simulink model "comparison_simulator"  (R2025b)
settings: Solver=VariableStepAuto  StartTime=0.0  StopTime=1000  RelTol=1e-3
values from neighbouring files (symbols this model uses):
  FO_PI = minreal(kp_FO + kp_FO*ki_FO*tf(1,[1 0])*s_alfa1, 0.1)    [controller_design.m]
  Hc_GT = minreal((1/H_p) * (Ho_GT / (1-Ho_GT)))    [controller_design.m]
  Hc_PI = minreal(ki_PI * (1 + tf(1, [Ti_PI 0])))    [controller_design.m]
  Rc_IMC = minreal(Hc_IMC / minreal(1 - Hc_IMC * H_p))    [controller_design.m]
undefined symbols (not defined in the file or in its folder): MAP_model, paramGrecoMAP
libraries: slpidlib x1
settings Model: Creator=ciuba  LastModifiedBy=ciuba

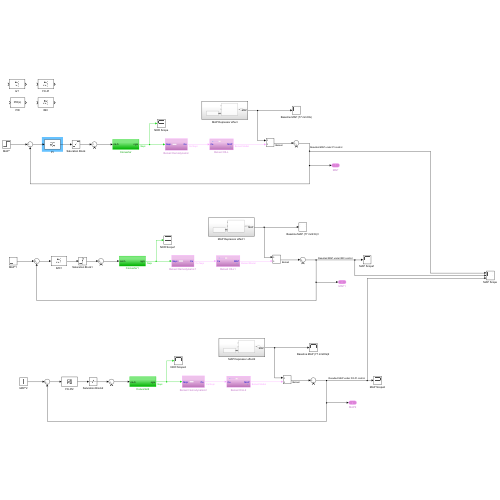
[thumbnail: Simulink's stored preview of the top-level diagram]
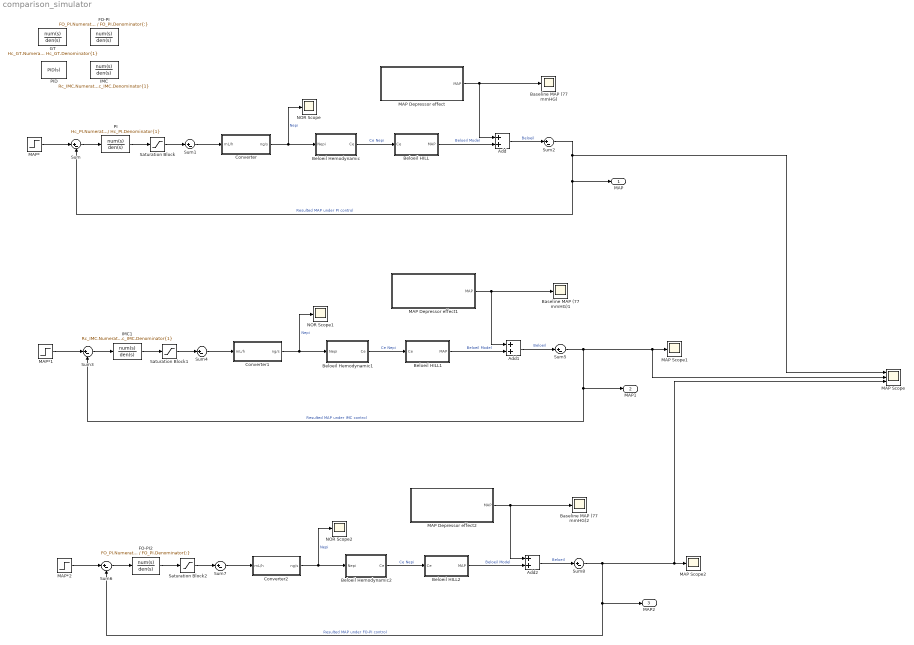
== system comparison_simulator ==
  Add : Sum
  Add1 : Sum
  Add2 : Sum
  Baseline MAP (77 mmHG) : Scope
      settings: ActiveDisplayYMinimum=-1  ActiveDisplayYMaximum=1  DataLoggingVariableName=ScopeData6
  Baseline MAP (77 mmHG)1 : Scope
      settings: ActiveDisplayYMinimum=-1  ActiveDisplayYMaximum=1
  Baseline MAP (77 mmHG)2 : Scope
      settings: ActiveDisplayYMinimum=-1  ActiveDisplayYMaximum=1  DataLoggingVariableName=ScopeData3
  Beloeil HILL : Subsystem
  Beloeil HILL1 : Subsystem
  Beloeil HILL2 : Subsystem
  Beloeil Hemodynamic : Subsystem
  Beloeil Hemodynamic1 : Subsystem
  Beloeil Hemodynamic2 : Subsystem
  Converter : Subsystem
  Converter1 : Subsystem
  Converter2 : Subsystem
  FO-PI : TransferFcn  Numerator=FO_PI.Numerator{:}  Denominator=FO_PI.Denominator{:}
  FO-PI2 : TransferFcn  Numerator=FO_PI.Numerator{:}  Denominator=FO_PI.Denominator{:}
  GT : TransferFcn  Numerator=Hc_GT.Numerator{1}  Denominator=Hc_GT.Denominator{1}
  IMC : TransferFcn  Numerator=Rc_IMC.Numerator{1}  Denominator=Rc_IMC.Denominator{1}
  IMC1 : TransferFcn  Numerator=Rc_IMC.Numerator{1}  Denominator=Rc_IMC.Denominator{1}
  MAP Depressor effect : Subsystem
  MAP Depressor effect1 : Subsystem
  MAP Depressor effect2 : Subsystem
  MAP Scope : Scope  NumInputPorts=3
      settings: ActiveDisplayYMinimum=75.156439251217392  ActiveDisplayYMaximum=93.5920467390435  DataLoggingVariableName=ScopeData4
  MAP Scope1 : Scope
      settings: ActiveDisplayYMinimum=75.156363433588581  ActiveDisplayYMaximum=93.592729097702758
  MAP Scope2 : Scope
      settings: ActiveDisplayYMinimum=75.156363433588581  ActiveDisplayYMaximum=93.592729097702758  DataLoggingVariableName=ScopeData5
  MAP* : Step  After=90  SampleTime=0
  MAP*1 : Step  After=90  SampleTime=0
  MAP*2 : Step  After=90  SampleTime=0
  NOR Scope : Scope
      settings: ActiveDisplayYMinimum=-446.02327911069489  ActiveDisplayYMaximum=4014.2095119962551  DataLoggingVariableName=ScopeData10  DataLoggingSaveFormat=Array
  NOR Scope1 : Scope
      settings: ActiveDisplayYMinimum=-446.02327911069489  ActiveDisplayYMaximum=4014.2095119962551  DataLoggingVariableName=ScopeData2  DataLoggingSaveFormat=Array
  NOR Scope2 : Scope
      settings: ActiveDisplayYMinimum=-446.02327911069489  ActiveDisplayYMaximum=4014.2095119962551  DataLoggingVariableName=ScopeData7  DataLoggingSaveFormat=Array
  PI : TransferFcn  Numerator=Hc_PI.Numerator{1}  Denominator=Hc_PI.Denominator{1}
  PID : slpidlib/PID Controller  Controller=PID  Form=Parallel  TimeDomain=Continuous-time  UseExternalTs=off  SampleTime=-1  IntegratorMethod=Forward Euler  FilterMethod=Forward Euler  ControllerParametersSource=internal  P=35.6  I=4.93  UseKiTs=off  D=64.4  UseExternalDerivativeSource=off  N=100  UseFilter=on  TunerSelectOption=Transfer Function Based (PID Tuner App)  InitialConditionSource=internal  InitialConditionForIntegrator=0  InitialConditionForFilter=0  DifferentiatorICPrevScaledInput=0  ExternalReset=none  TrackingMode=off  Kt=1  LimitOutput=off  SatLimitsSource=internal  UpperSaturationLimit=inf  LowerSaturationLimit=-inf  LinearizeAsGain=on  AntiWindupMode=none  Kb=1  LimitIntegrator=off  UpperIntegratorSaturationLimit=inf  LowerIntegratorSaturationLimit=-inf  POutMin=[]  POutMax=[]  IOutMin=[]  IOutMax=[]  DOutMin=[]  DOutMax=[]  NOutMin=[]  NOutMax=[]  SumOutMin=[]  SumOutMax=[]  SaturationOutMin=[]  SaturationOutMax=[]  PParamMin=[]  PParamMax=[]  IParamMin=[]  IParamMax=[]  DParamMin=[]  DParamMax=[]  NParamMin=[]  NParamMax=[]  KbParamMin=[]  KbParamMax=[]  KtParamMin=[]  KtParamMax=[]  KbOutMin=[]  KbOutMax=[]  KtOutMin=[]  KtOutMax=[]  IntegratorOutMin=[]  IntegratorOutMax=[]  FilterOutMin=[]  FilterOutMax=[]  SumI1OutMin=[]  SumI1OutMax=[]  SumI2OutMin=[]  SumI2OutMax=[]  SumI3OutMin=[]  SumI3OutMax=[]  SumI4OutMin=[]  SumI4OutMax=[]  SumDOutMin=[]  SumDOutMax=[]  DifferentiatorOutMin=[]  DifferentiatorOutMax=[]  FilterDiffOutCoefMin=[]  FilterDiffOutCoefMax=[]  ReciprocalOutMin=[]  ReciprocalOutMax=[]  SumDenOutMin=[]  SumDenOutMax=[]  SumNumOutMin=[]  SumNumOutMax=[]  DivideOutMin=[]  DivideOutMax=[]  UdiffTsProdOutMin=[]  UdiffTsProdOutMax=[]  NTsProdOutMin=[]  NTsProdOutMax=[]  UintegralTsProdOutMin=[]  UintegralTsProdOutMax=[]  UngainTsProdOutMin=[]  UngainTsProdOutMax=[]  ClampingZeroOutDataTypeStr=Inherit: Inherit via back propagation  ClampingZeroOutMin=[]  ClampingZeroOutMax=[]  FilterDenConstantOutDataTypeStr=Inherit: Inherit via back propagation  FilterDenConstantOutMin=[]  FilterDenConstantOutMax=[]  PCopyOutDataTypeStr=Inherit: Inherit via back propagation  PCopyOutMin=[]  PCopyOutMax=[]  NCopyOutDataTypeStr=Inherit: Inherit via back propagation  NCopyOutMin=[]  NCopyOutMax=[]  IntegratorContinuousStateAttributes=''  IntegratorStateMustResolveToSignalObject=off  IntegratorRTWStateStorageClass=Auto  FilterContinuousStateAttributes=''  FilterStateMustResolveToSignalObject=off  FilterRTWStateStorageClass=Auto  ParallelPVariant=InternalParameters  IdealPVariant=Disabled  IVariant=InternalParameters  DVariant=InternalParameters  IntegratorVariant=Continuous  SatVariant=Disabled  AWVariant=Passthrough  PCopyVariant=Disabled  TRVariant=Disabled  FdbkBlocksVariant=Forward  IdealPFdbkVariant=Disabled  SatFdbkVariant=Disabled  DerivativeFilterVariant=ContFilter  NVariant=InternalParameters  NCopyVariant=Disabled  FilterICVariant=InternalICsFilter  IntegratorICVariant=InternalICs  ExternalResetVariant=Disabled  TRSumVariant=Passthrough  SumFdbkVariant=Disabled  SumVariant=Sum_PID  TsampFilterVariant=InternalTs  TsampNgainVariant=Passthrough  TsampIntegralVariant=Disabled_SignalSpec  ExternalSaturationOutDataTypeStr=Inherit: Same as second input  DerivativeSourceVariant=ErrorSignal  PreIntVariant=InternalPreInt
  Saturation Block : Saturate  UpperLimit=5000  LowerLimit=0
  Saturation Block1 : Saturate  UpperLimit=5000  LowerLimit=0
  Saturation Block2 : Saturate  UpperLimit=5000  LowerLimit=0
  Sum{,1..8} (9 alike) : Sum  Inputs=|+-
  MAP : Outport
  MAP1 : Outport  Port=2
  MAP2 : Outport  Port=3
  wires:
  Sum/1 -> PI/1
  PI/1 -> Saturation Block/1
  Beloeil HILL/1(MAP) -> Add/2  "Beloeil Model"
  Sum1/1 -> Converter/1(mL/h)
  Converter/1(ng/s) -> NOR Scope/1, Beloeil Hemodynamic/1(Nepi)  "Nepi"
  Beloeil Hemodynamic/1(Ce) -> Beloeil HILL/1(Ce)  "Ce Nepi"
  Sum2/1 -> Sum/2, MAP/1, MAP Scope/1  "Resulted MAP under PI control"
  MAP*/1 -> Sum/1
  Add/1 -> Sum2/1  "Beloeil"
  Saturation Block/1 -> Sum1/1
  MAP Depressor effect/1(MAP) -> Add/1, Baseline MAP (77 mmHG)/1
  Sum3/1 -> IMC1/1
  IMC1/1 -> Saturation Block1/1
  Beloeil HILL1/1(MAP) -> Add1/2  "Beloeil Model"
  Sum4/1 -> Converter1/1(mL/h)
  Converter1/1(ng/s) -> NOR Scope1/1, Beloeil Hemodynamic1/1(Nepi)  "Nepi"
  Beloeil Hemodynamic1/1(Ce) -> Beloeil HILL1/1(Ce)  "Ce Nepi"
  Sum5/1 -> Sum3/2, MAP1/1, MAP Scope/2, MAP Scope1/1  "Resulted MAP under IMC control"
  MAP*1/1 -> Sum3/1
  Add1/1 -> Sum5/1  "Beloeil"
  Saturation Block1/1 -> Sum4/1
  MAP Depressor effect1/1(MAP) -> Add1/1, Baseline MAP (77 mmHG)1/1
  Sum6/1 -> FO-PI2/1
  FO-PI2/1 -> Saturation Block2/1
  Beloeil HILL2/1(MAP) -> Add2/2  "Beloeil Model"
  Sum7/1 -> Converter2/1(mL/h)
  Converter2/1(ng/s) -> NOR Scope2/1, Beloeil Hemodynamic2/1(Nepi)  "Nepi"
  Beloeil Hemodynamic2/1(Ce) -> Beloeil HILL2/1(Ce)  "Ce Nepi"
  Sum8/1 -> Sum6/2, MAP2/1, MAP Scope/3, MAP Scope2/1  "Resulted MAP under FO-PI control"
  MAP*2/1 -> Sum6/1
  Add2/1 -> Sum8/1  "Beloeil"
  Saturation Block2/1 -> Sum7/1
  MAP Depressor effect2/1(MAP) -> Add2/1, Baseline MAP (77 mmHG)2/1

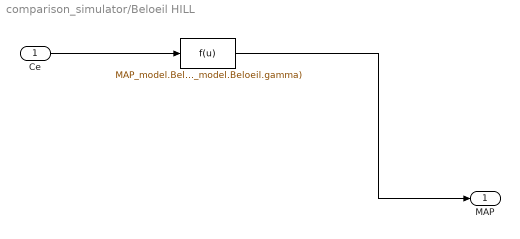
== system comparison_simulator/Beloeil HILL ==
  Ce : Inport
  " " : Fcn  Expr=MAP_model.Beloeil.Emax * (u^MAP_model.Beloeil.gamma) / (MAP_model.Beloeil.EC50^MAP_model.Beloeil.gamma+u^MAP_model.Beloeil.gamma)
  MAP : Outport
  wires:
  " "/1 -> MAP/1
  Ce/1 -> " "/1

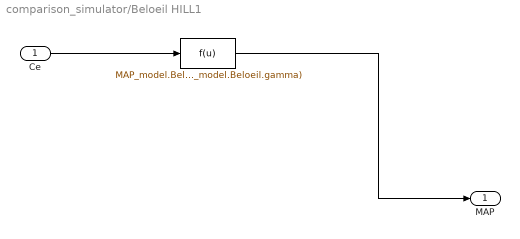
== system comparison_simulator/Beloeil HILL1 ==
  Ce : Inport
  " " : Fcn  Expr=MAP_model.Beloeil.Emax * (u^MAP_model.Beloeil.gamma) / (MAP_model.Beloeil.EC50^MAP_model.Beloeil.gamma+u^MAP_model.Beloeil.gamma)
  MAP : Outport
  wires:
  " "/1 -> MAP/1
  Ce/1 -> " "/1

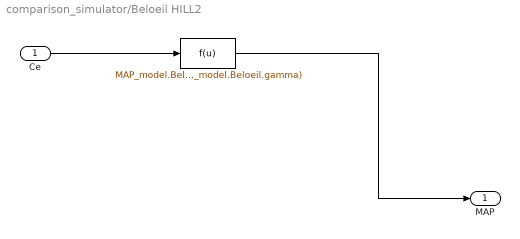
== system comparison_simulator/Beloeil HILL2 ==
  Ce : Inport
  " " : Fcn  Expr=MAP_model.Beloeil.Emax * (u^MAP_model.Beloeil.gamma) / (MAP_model.Beloeil.EC50^MAP_model.Beloeil.gamma+u^MAP_model.Beloeil.gamma)
  MAP : Outport
  wires:
  " "/1 -> MAP/1
  Ce/1 -> " "/1

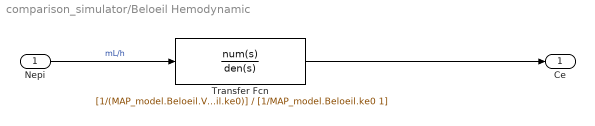
== system comparison_simulator/Beloeil Hemodynamic ==
  Nepi : Inport
  Transfer Fcn : TransferFcn  Numerator=[1/(MAP_model.Beloeil.Vd*MAP_model.Beloeil.ke0)]  Denominator=[1/MAP_model.Beloeil.ke0 1]
  Ce : Outport
  wires:
  Nepi/1 -> Transfer Fcn/1  "mL/h"
  Transfer Fcn/1 -> Ce/1

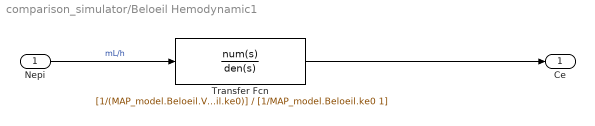
== system comparison_simulator/Beloeil Hemodynamic1 ==
  Nepi : Inport
  Transfer Fcn : TransferFcn  Numerator=[1/(MAP_model.Beloeil.Vd*MAP_model.Beloeil.ke0)]  Denominator=[1/MAP_model.Beloeil.ke0 1]
  Ce : Outport
  wires:
  Nepi/1 -> Transfer Fcn/1  "mL/h"
  Transfer Fcn/1 -> Ce/1

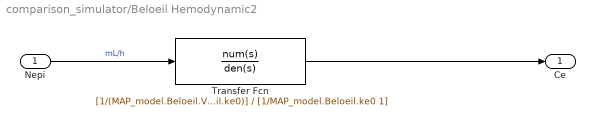
== system comparison_simulator/Beloeil Hemodynamic2 ==
  Nepi : Inport
  Transfer Fcn : TransferFcn  Numerator=[1/(MAP_model.Beloeil.Vd*MAP_model.Beloeil.ke0)]  Denominator=[1/MAP_model.Beloeil.ke0 1]
  Ce : Outport
  wires:
  Nepi/1 -> Transfer Fcn/1  "mL/h"
  Transfer Fcn/1 -> Ce/1

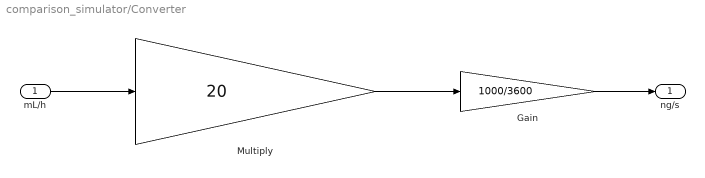
== system comparison_simulator/Converter ==
  mL/h : Inport
  Gain : Gain  Gain=1000/3600
  Multiply : Gain  Gain=20
  ng/s : Outport
  wires:
  Gain/1 -> ng/s/1
  Multiply/1 -> Gain/1
  mL/h/1 -> Multiply/1

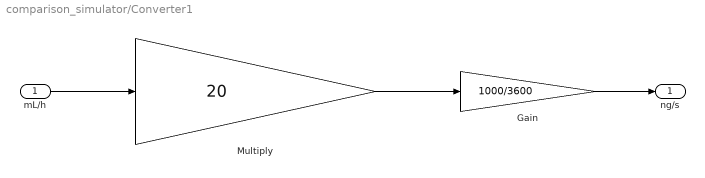
== system comparison_simulator/Converter1 ==
  mL/h : Inport
  Gain : Gain  Gain=1000/3600
  Multiply : Gain  Gain=20
  ng/s : Outport
  wires:
  Gain/1 -> ng/s/1
  Multiply/1 -> Gain/1
  mL/h/1 -> Multiply/1

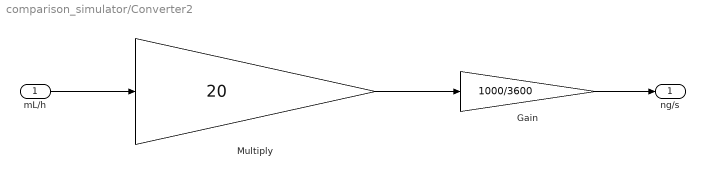
== system comparison_simulator/Converter2 ==
  mL/h : Inport
  Gain : Gain  Gain=1000/3600
  Multiply : Gain  Gain=20
  ng/s : Outport
  wires:
  Gain/1 -> ng/s/1
  Multiply/1 -> Gain/1
  mL/h/1 -> Multiply/1

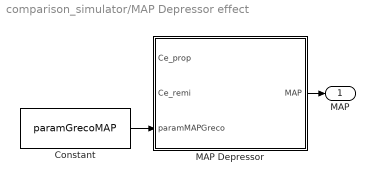
== system comparison_simulator/MAP Depressor effect ==
  Constant : Constant  Value=paramGrecoMAP  OutDataTypeStr=Bus: GrecoMAPBus
  MAP Depressor : MATLAB Function  TreatAsAtomicUnit=on
  MAP : Outport
  wires:
  MAP Depressor/1(MAP) -> MAP/1
  Constant/1 -> MAP Depressor/3(paramMAPGreco)

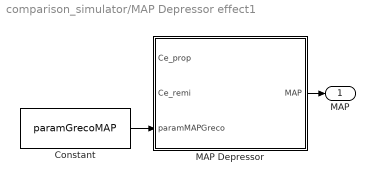
== system comparison_simulator/MAP Depressor effect1 ==
  Constant : Constant  Value=paramGrecoMAP  OutDataTypeStr=Bus: GrecoMAPBus
  MAP Depressor : MATLAB Function  TreatAsAtomicUnit=on
  MAP : Outport
  wires:
  MAP Depressor/1(MAP) -> MAP/1
  Constant/1 -> MAP Depressor/3(paramMAPGreco)

== system comparison_simulator/MAP Depressor effect2 ==
  Constant : Constant  Value=paramGrecoMAP  OutDataTypeStr=Bus: GrecoMAPBus
  MAP Depressor : MATLAB Function  TreatAsAtomicUnit=on
  MAP : Outport
  wires:
  MAP Depressor/1(MAP) -> MAP/1
  Constant/1 -> MAP Depressor/3(paramMAPGreco)

== matlab function comparison_simulator/MAP Depressor effect/MAP Depressor ==
  data: Ce_prop input; MAP output; Ce_remi input; paramMAPGreco input
function MAP = MAP_Greco(Ce_prop, Ce_remi, paramMAPGreco)    
    % Extract parameters from bus
    C50P   = paramMAPGreco.Prop.C50;    % Propofol EC50 (μg/mL)
    gammaP = paramMAPGreco.Prop.gamma;  % Propofol Hill
    C50R   = paramMAPGreco.Remi.C50;    % Remifentanil EC50 (ng/mL)
    gammaR = paramMAPGreco.Remi.gamma;  % Remifentanil Hill
    alpha  = paramMAPGreco.Interaction.alpha;  % Synergy parameter
    Emax   = paramMAPGreco.Interaction.Emax;   % Max MAP depression (mmHg)
    MAP0   = paramMAPGreco.Interaction.MAP0;   % Baseline MAP (mmHg)
    
    % Compute normalized concentrations
    X = (Ce_prop / C50P)^gammaP;
    Y = (Ce_remi / C50R)^gammaR;
    
    % Numerator/denominator as per Greco response surface
    numerator   = X + Y + alpha * X * Y;
    denominator = 1 + X + Y + alpha * X * Y;
    MAP_depr    = Emax * numerator / denominator;
    
    % Net MAP (subtract depressant effect from baseline)
    MAP = MAP0 - MAP_depr;
end

== matlab function comparison_simulator/MAP Depressor effect1/MAP Depressor ==
  data: Ce_prop input; MAP output; Ce_remi input; paramMAPGreco input
function MAP = MAP_Greco(Ce_prop, Ce_remi, paramMAPGreco)    
    % Extract parameters from bus
    C50P   = paramMAPGreco.Prop.C50;    % Propofol EC50 (μg/mL)
    gammaP = paramMAPGreco.Prop.gamma;  % Propofol Hill
    C50R   = paramMAPGreco.Remi.C50;    % Remifentanil EC50 (ng/mL)
    gammaR = paramMAPGreco.Remi.gamma;  % Remifentanil Hill
    alpha  = paramMAPGreco.Interaction.alpha;  % Synergy parameter
    Emax   = paramMAPGreco.Interaction.Emax;   % Max MAP depression (mmHg)
    MAP0   = paramMAPGreco.Interaction.MAP0;   % Baseline MAP (mmHg)
    
    % Compute normalized concentrations
    X = (Ce_prop / C50P)^gammaP;
    Y = (Ce_remi / C50R)^gammaR;
    
    % Numerator/denominator as per Greco response surface
    numerator   = X + Y + alpha * X * Y;
    denominator = 1 + X + Y + alpha * X * Y;
    MAP_depr    = Emax * numerator / denominator;
    
    % Net MAP (subtract depressant effect from baseline)
    MAP = MAP0 - MAP_depr;
end

== matlab function comparison_simulator/MAP Depressor effect2/MAP Depressor ==
  data: Ce_prop input; MAP output; Ce_remi input; paramMAPGreco input
function MAP = MAP_Greco(Ce_prop, Ce_remi, paramMAPGreco)    
    % Extract parameters from bus
    C50P   = paramMAPGreco.Prop.C50;    % Propofol EC50 (μg/mL)
    gammaP = paramMAPGreco.Prop.gamma;  % Propofol Hill
    C50R   = paramMAPGreco.Remi.C50;    % Remifentanil EC50 (ng/mL)
    gammaR = paramMAPGreco.Remi.gamma;  % Remifentanil Hill
    alpha  = paramMAPGreco.Interaction.alpha;  % Synergy parameter
    Emax   = paramMAPGreco.Interaction.Emax;   % Max MAP depression (mmHg)
    MAP0   = paramMAPGreco.Interaction.MAP0;   % Baseline MAP (mmHg)
    
    % Compute normalized concentrations
    X = (Ce_prop / C50P)^gammaP;
    Y = (Ce_remi / C50R)^gammaR;
    
    % Numerator/denominator as per Greco response surface
    numerator   = X + Y + alpha * X * Y;
    denominator = 1 + X + Y + alpha * X * Y;
    MAP_depr    = Emax * numerator / denominator;
    
    % Net MAP (subtract depressant effect from baseline)
    MAP = MAP0 - MAP_depr;
end
